simulink model "SaturationAndDeadzoneExample"  (Simulink 9.0)
settings: Solver=VariableStepAuto  StartTime=0.0  StopTime=3  RelTol=1e-3
libraries: simulink x1
settings Model: Creator=efrem  LastModifiedBy=efrem
settings DataIOCC: SaveFormat=Dataset
settings OptimizationCC: LifeSpan=auto
settings DebuggingCC: UnderspecifiedInitializationDetection=Simplified  MergeDetectMultiDrivingBlocksExec=error  SFUnexpectedBacktrackingDiag=error  SFNoUnconditionalDefaultTransitionDiag=error  SFExecutionAtInitializationDiag=warning
settings HardwareCC: ProdBitPerPointer=64  ProdBitPerSizeT=64  ProdBitPerPtrDiffT=64  ProdLargestAtomicFloat=Float  ProdIntDivRoundTo=Zero  ProdEndianess=LittleEndian  ProdWordSize=64  ProdHWDeviceType=Intel->x86-64 (Windows64)
settings ModelReferenceCC: PropagateSignalLabelsOutOfModel=on
settings CodeAppCC: StateflowObjectComments=off
settings GRTTargetCC: TargetLangStandard=C99 (ISO)
settings ConfigComp: CovMetricSettings=dwe  CovHtmlReporting=off  CovSaveCumulativeToWorkspaceVar=off  CovSaveSingleToWorkspaceVar=off  CovExternalEMLEnable=on

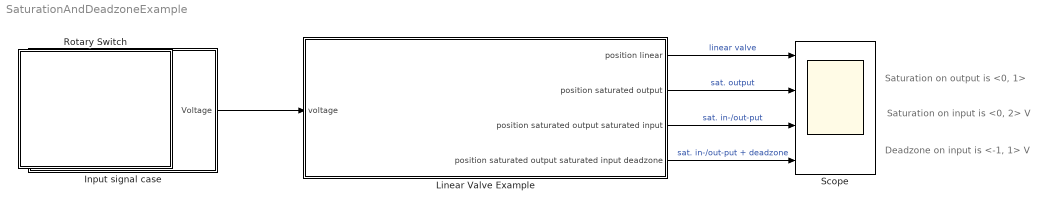
== system SaturationAndDeadzoneExample ==
  note: Saturation on output is <0, 1>
  note: Saturation on input is <0, 2> V
  note: Deadzone on input is <-1, 1> V
  Input signal case : Subsystem  mask{signal_case=2}
      mask prompts: signal_case "Signal type"
  Linear Valve Example : Subsystem
  Rotary Switch : Subsystem  DialogController=hmiCreateDDGDialog  DialogControllerArgs=DataTag0  IsWebBlock=on  mask(MWDashboardBlock){webBlockId=d06cba31-a511-4312-a727-2ae7a5e97082, webBlockType=discreteknob, ShowInLibBrowser=on, ShowInitialText=on, HMISrcModelName=SaturationAndDeadzoneExample}
      mask prompts: webBlockId "WebBlock Id"; webBlockType "WebBlock Type"; HMISrcModelName "Source Model"
      mask help: Set value to tune parameters or variables.
      mask Help: helpview([docroot '/mapfiles/simulink.map'], 'hmi_rotary_switch')
      mask Display:
      | if strcmp(get_param(bdroot(gcb),'BlockDiagramType'),'library')
      |  image([(matlabroot) '/toolbox/simulink/hmi/icons/DiscreteKnob.png'])
      | end
  Scope : Scope  NumInputPorts=4
  wires:
  Linear Valve Example/1(position linear) -> Scope/1  "linear valve"
  Linear Valve Example/2(position saturated output) -> Scope/2  "sat. output"
  Linear Valve Example/3(position saturated output saturated input) -> Scope/3  "sat. in-/out-put"
  Linear Valve Example/4(position saturated output saturated input deadzone) -> Scope/4  "sat. in-/out-put + deadzone"
  Input signal case/1(Voltage) -> Linear Valve Example/1("voltage ")

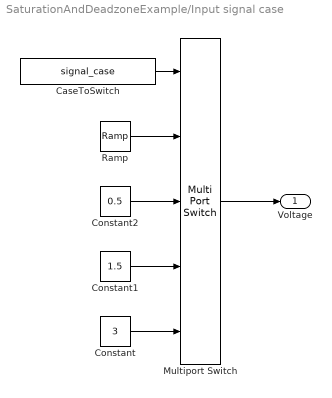
== system SaturationAndDeadzoneExample/Input signal case ==
  CaseToSwitch : Constant  Value=signal_case
  Constant : Constant  Value=3
  Constant1 : Constant  Value=1.5
  Constant2 : Constant  Value=0.5
  Multiport Switch : MultiPortSwitch  Inputs=4
  Ramp : simulink/Sources/Ramp  slope=2  start=0  X0=0
  Voltage : Outport
  wires:
  Constant2/1 -> Multiport Switch/3
  Constant/1 -> Multiport Switch/5
  Constant1/1 -> Multiport Switch/4
  CaseToSwitch/1 -> Multiport Switch/1
  Multiport Switch/1 -> Voltage/1
  Ramp/1 -> Multiport Switch/2

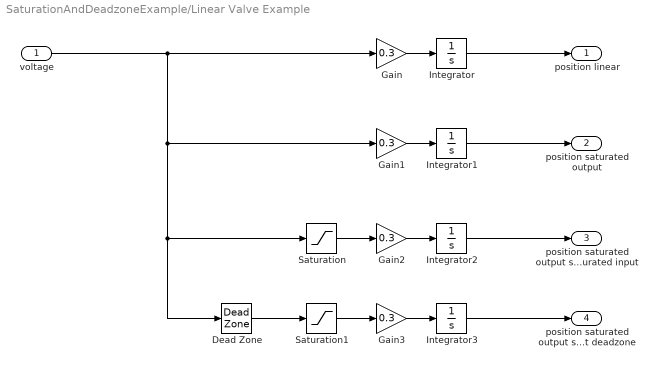
== system SaturationAndDeadzoneExample/Linear Valve Example ==
  "voltage " : Inport
  Dead Zone : DeadZone  LowerValue=-1  UpperValue=1
  Gain{,1..3} (4 alike) : Gain  Gain=0.3
  Integrator : Integrator
  Integrator1 : Integrator  LimitOutput=on  UpperSaturationLimit=1  LowerSaturationLimit=0
  Integrator2 : Integrator  LimitOutput=on  UpperSaturationLimit=1  LowerSaturationLimit=0
  Integrator3 : Integrator  LimitOutput=on  UpperSaturationLimit=1  LowerSaturationLimit=0
  Saturation : Saturate  UpperLimit=2  LowerLimit=0
  Saturation1 : Saturate  UpperLimit=2  LowerLimit=0
  position linear : Outport
  position saturated output : Outport  Port=2
  position saturated output saturated input : Outport  Port=3
  position saturated output saturated input deadzone : Outport  Port=4
  wires:
  Integrator/1 -> position linear/1
  Saturation/1 -> Gain2/1
  Saturation1/1 -> Gain3/1
  Integrator1/1 -> position saturated output/1
  Integrator2/1 -> position saturated output saturated input/1
  "voltage "/1 -> Gain1/1, Dead Zone/1, Saturation/1, Gain/1
  Integrator3/1 -> position saturated output saturated input deadzone/1
  Gain/1 -> Integrator/1
  Gain1/1 -> Integrator1/1
  Gain2/1 -> Integrator2/1
  Gain3/1 -> Integrator3/1
  Dead Zone/1 -> Saturation1/1

== system SaturationAndDeadzoneExample/Rotary Switch ==
